simulink model "Guidance_Equations"  (R2013a)
settings: Solver=ode4  StartTime=0.0  StopTime=10.0  FixedStep=0.0001  RelTol=1e-3
settings Model: Creator=Ibrahim_B92  LastModifiedBy=Ibrahim_B92

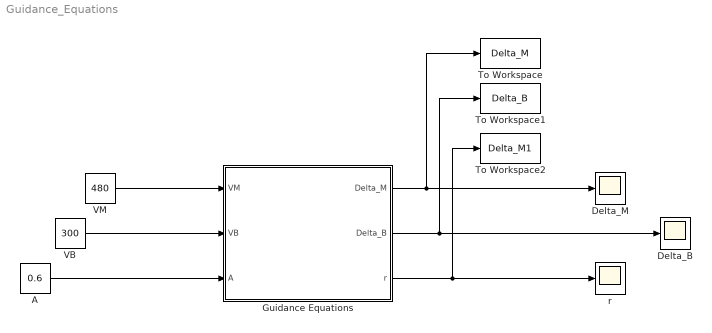
== system Guidance_Equations ==
  A : Constant  Value=0.6
  Delta_B : Scope
  Delta_M : Scope
  Guidance Equations : Subsystem
  To Workspace : ToWorkspace  VariableName=Delta_M  SampleTime=-1
  To Workspace1 : ToWorkspace  VariableName=Delta_B  SampleTime=-1
  To Workspace2 : ToWorkspace  VariableName=Delta_M1  SampleTime=-1  SaveFormat=Timeseries
  VB : Constant  Value=300
  VM : Constant  Value=480
  r : Scope
      settings: SaveName=ScopeData2
  wires:
  VM/1 -> Guidance Equations/1(VM)
  VB/1 -> Guidance Equations/2(VB)
  Guidance Equations/1(Delta_M) -> Delta_M/1, To Workspace/1
  Guidance Equations/2(Delta_B) -> Delta_B/1, To Workspace1/1
  Guidance Equations/3(r) -> To Workspace2/1, r/1
  A/1 -> Guidance Equations/3(A)

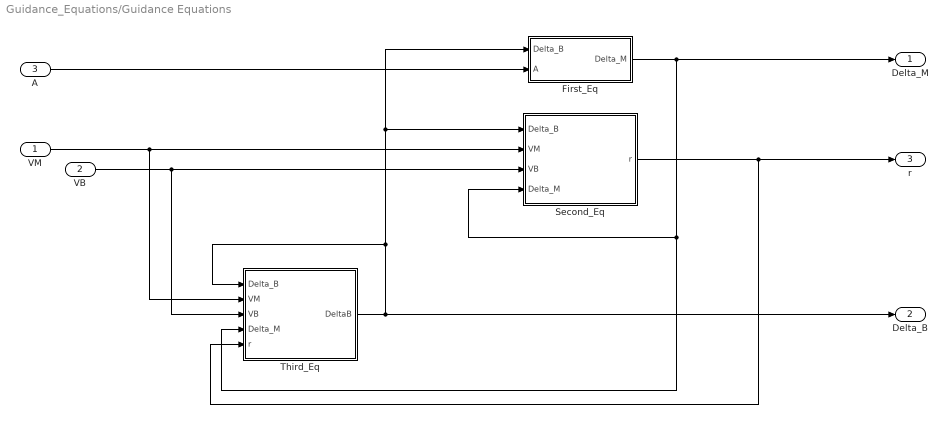
== system Guidance_Equations/Guidance Equations ==
  VM : Inport
  VB : Inport  Port=2
  A : Inport  Port=3
  First_Eq : Subsystem
  Second_Eq : Subsystem
  Third_Eq : Subsystem
  Delta_M : Outport
  Delta_B : Outport  Port=2
  r : Outport  Port=3
  wires:
  Third_Eq/1(DeltaB) -> Second_Eq/1(Delta_B), First_Eq/1(Delta_B), Third_Eq/1(Delta_B), Delta_B/1
  First_Eq/1(Delta_M) -> Delta_M/1, Third_Eq/4(Delta_M), Second_Eq/4(Delta_M)
  VM/1 -> Third_Eq/2(VM), Second_Eq/2(VM)
  VB/1 -> Third_Eq/3(VB), Second_Eq/3(VB)
  Second_Eq/1(r) -> Third_Eq/5(r), r/1
  A/1 -> First_Eq/2(A)

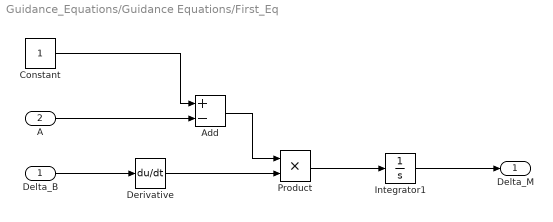
== system Guidance_Equations/Guidance Equations/First_Eq ==
  Delta_B : Inport
  A : Inport  Port=2
  Add : Sum  Inputs=+-
  Constant : Constant
  Derivative : Derivative
  Integrator1 : Integrator
  Product : Product
  Delta_M : Outport
  wires:
  Delta_B/1 -> Derivative/1
  Derivative/1 -> Product/2
  Product/1 -> Integrator1/1
  Integrator1/1 -> Delta_M/1
  A/1 -> Add/2
  Constant/1 -> Add/1
  Add/1 -> Product/1

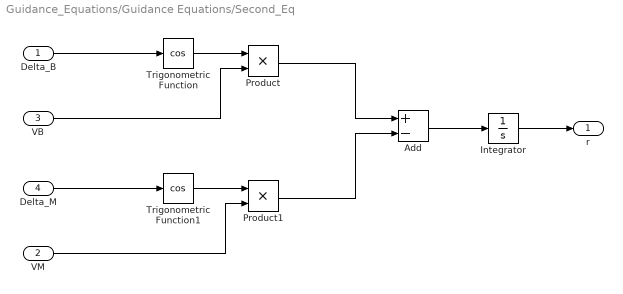
== system Guidance_Equations/Guidance Equations/Second_Eq ==
  Delta_B : Inport
  VM : Inport  Port=2
  VB : Inport  Port=3
  Delta_M : Inport  Port=4
  Add : Sum  Inputs=+-
  Integrator : Integrator
  Product : Product
  Product1 : Product
  Trigonometric Function : Trigonometry  Operator=cos
  Trigonometric Function1 : Trigonometry  Operator=cos
  r : Outport
  wires:
  Delta_B/1 -> Trigonometric Function/1
  Delta_M/1 -> Trigonometric Function1/1
  VB/1 -> Product/2
  Trigonometric Function/1 -> Product/1
  Trigonometric Function1/1 -> Product1/1
  VM/1 -> Product1/2
  Product/1 -> Add/1
  Product1/1 -> Add/2
  Add/1 -> Integrator/1
  Integrator/1 -> r/1

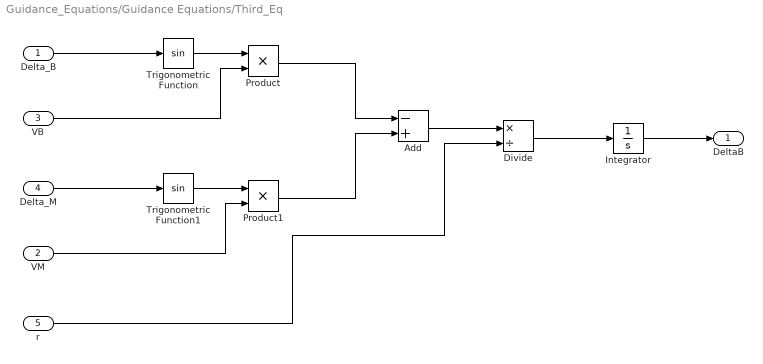
== system Guidance_Equations/Guidance Equations/Third_Eq ==
  Delta_B : Inport
  VM : Inport  Port=2
  VB : Inport  Port=3
  Delta_M : Inport  Port=4
  r : Inport  Port=5
  Add : Sum  Inputs=-+
  Divide : Product  Inputs=*/
  Integrator : Integrator
  Product : Product
  Product1 : Product
  Trigonometric Function : Trigonometry
  Trigonometric Function1 : Trigonometry
  DeltaB : Outport
  wires:
  Delta_B/1 -> Trigonometric Function/1
  Delta_M/1 -> Trigonometric Function1/1
  VB/1 -> Product/2
  Trigonometric Function/1 -> Product/1
  Trigonometric Function1/1 -> Product1/1
  VM/1 -> Product1/2
  Product/1 -> Add/1
  Product1/1 -> Add/2
  Add/1 -> Divide/1
  Divide/1 -> Integrator/1
  Integrator/1 -> DeltaB/1
  r/1 -> Divide/2
